simulink model "sparse_parameter_test_simulink"  (R2023a)
settings: Solver=ode45  StartTime=0.0  StopTime=0.1  RelTol=1e-3
undefined symbols (not defined in the file or in its folder): input_update_port_first8, input_update_port_p4243
settings Model: Creator=oj  LastModifiedBy=oj
settings SolverCC: AlgebraicLoopSolver=TrustRegion
settings DataIOCC: SaveFormat=StructureWithTime
settings OptimizationCC: LifeSpan=inf
settings DebuggingCC: FcnCallInpInsideContextMsg=warning  UnconnectedInputMsg=warning  UnconnectedOutputMsg=warning  UnconnectedLineMsg=warning  SFExecutionAtInitializationDiag=none  ArithmeticOperatorsInVariantConditions=warning
settings HardwareCC: ProdBitPerSizeT=32  ProdBitPerPtrDiffT=32  ProdWordSize=32  ProdHWDeviceType=Specified
settings SFSimCC: CustomCodeUndefinedFunction=UseInterfaceOnly
settings CodeAppCC: StateflowObjectComments=on

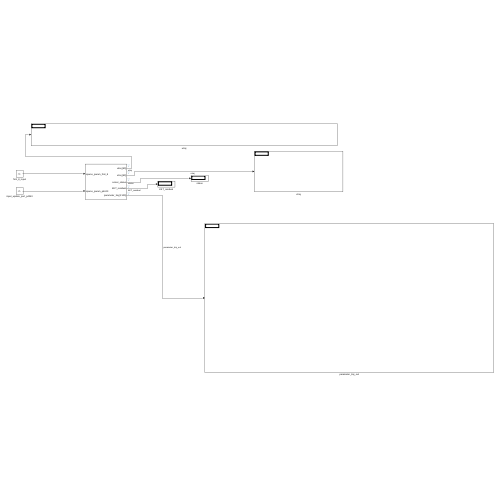
[thumbnail: Simulink's stored preview of the top-level diagram]
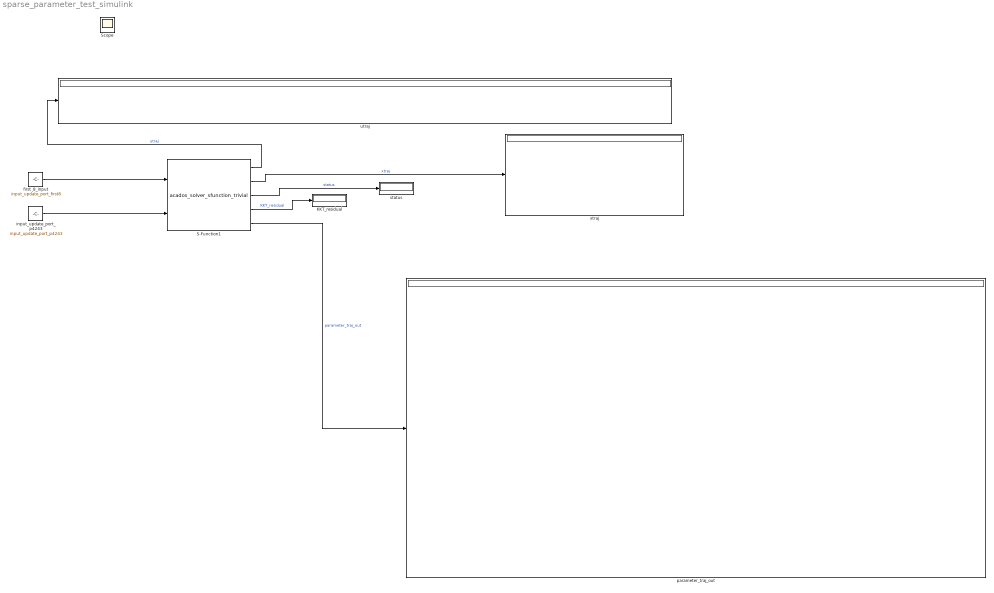
== system sparse_parameter_test_simulink ==
  KKT_residual : Display
  S-Function1 : S-Function  FunctionName=acados_solver_sfunction_trivial  SFunctionDeploymentMode=off  EnableBusSupport=off
      mask Display:
      | global sfun_input_names sfun_output_names
      | for i = 1:length(sfun_input_names)
      | 	port_label('input', i, sfun_input_names{i})
      | end
      | for i = 1:length(sfun_output_names)
      | 	port_label('output', i, sfun_output_names{i})
      | end
  first_8_input : Constant  Value=input_update_port_first8
  input_update_port_p4243 : Constant  Value=input_update_port_p4243
  parameter_traj_out : Display
  status : Display
  utraj : Display
  xtraj : Display
  Scope : Scope
  wires:
  S-Function1/3 -> status/1  "status"
  S-Function1/1 -> utraj/1  "utraj"
  S-Function1/2 -> xtraj/1  "xtraj"
  first_8_input/1 -> S-Function1/1
  S-Function1/5 -> parameter_traj_out/1  "parameter_traj_out"
  S-Function1/4 -> KKT_residual/1  "KKT_residual"
  input_update_port_p4243/1 -> S-Function1/2
